simulink model "ctrl_model_motor"  (R2018b)
settings: Solver=VariableStepAuto  StartTime=0.0  StopTime=10.0  RelTol=1e-3
undefined symbols (not defined in the file or in its folder): Bm, Il, Im, Km, La, Ra
settings Model: Creator=angel  LastModifiedBy=angel

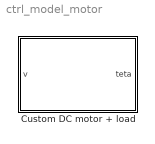
== system ctrl_model_motor ==
  Custom DC motor + load : Subsystem  ClipboardFcn=run('init_throttle.m')

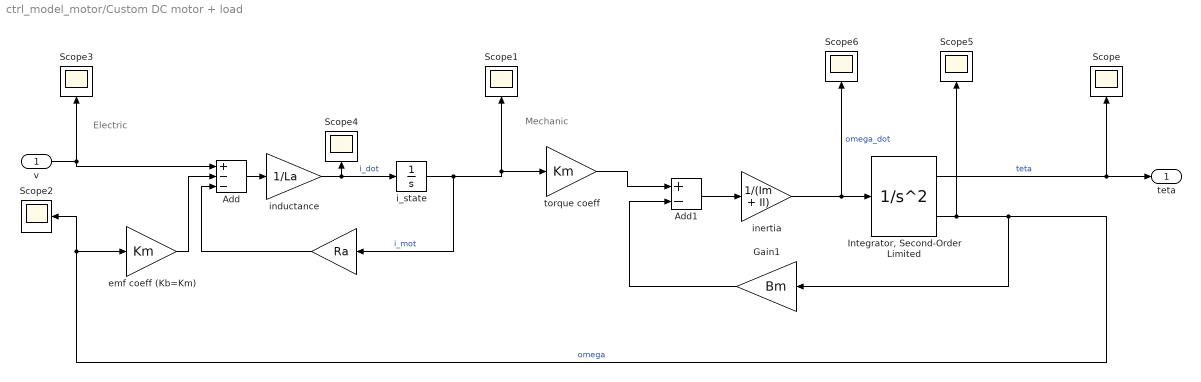
== system ctrl_model_motor/Custom DC motor + load ==
  note: Electric
  note: Mechanic
  v : Inport
  " " : Gain  Gain=Ra
  Add : Sum  Inputs=+--
  Add1 : Sum  Inputs=+-
  Gain1 : Gain  Gain=Bm
  "Integrator, Second-Order Limited" : SecondOrderIntegrator  UpperLimitX=1000  LowerLimitX=-1000  StateNameX='teta_state'  StateNameDXDT='omega_state'  ReinitDXDTwhenXreachesSaturation=on
  Scope{,1..6} (7 alike) : Scope
  "emf coeff (Kb=Km)    " : Gain  Gain=Km
  i_state : Integrator  LimitOutput=on  UpperSaturationLimit=1000  LowerSaturationLimit=-1000
  inductance : Gain  Gain=1/La
  inertia : Gain  Gain=1/(Im + Il)
  torque coeff : Gain  Gain=Km
  teta : Outport
  wires:
  Add1/1 -> inertia/1
  Gain1/1 -> Add1/2
  "Integrator, Second-Order Limited"/1 -> Scope/1, teta/1  "teta"
  "Integrator, Second-Order Limited"/2 -> Scope5/1, Scope2/1, "emf coeff (Kb=Km)    "/1, Gain1/1  "omega"
  inertia/1 -> "Integrator, Second-Order Limited"/1, Scope6/1  "omega_dot"
  i_state/1 -> " "/1, torque coeff/1, Scope1/1  "i_mot"
  v/1 -> Scope3/1, Add/1
  inductance/1 -> Scope4/1, i_state/1  "i_dot"
  " "/1 -> Add/3
  "emf coeff (Kb=Km)    "/1 -> Add/2
  Add/1 -> inductance/1
  torque coeff/1 -> Add1/1
